simulink model "CiEngineController"  (R2026b)
undefined symbols (not defined in the file): CtrlEcuTs
libraries: autolibengctrlr x1
settings Model: Creator=The MathWorks, Inc.  LastModifiedBy=The MathWorks, Inc.

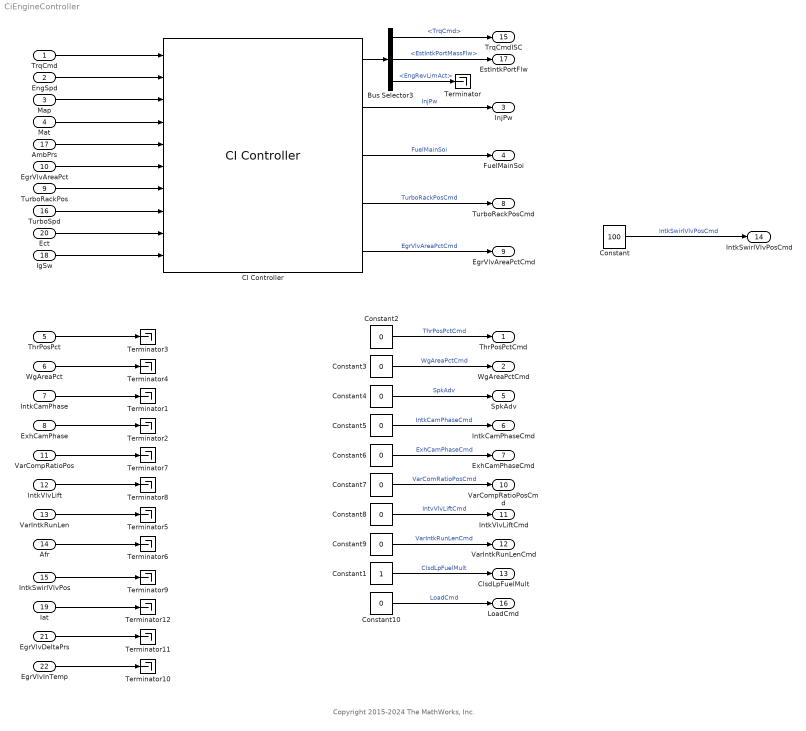
== system CiEngineController ==
  note: Copyright 2015-2024 The MathWorks, Inc.
  TrqCmd : Inport  OutDataTypeStr=double  Unit=N*m  PortDimensions=1
  EngSpd : Inport  Port=2  OutDataTypeStr=double  Unit=rpm  PortDimensions=1
  Map : Inport  Port=3  OutDataTypeStr=double  Unit=Pa  PortDimensions=1
  Mat : Inport  Port=4  OutDataTypeStr=double  Unit=K  PortDimensions=1
  ThrPosPct : Inport  Port=5  OutDataTypeStr=double  Unit=%  PortDimensions=1
  WgAreaPct : Inport  Port=6  OutDataTypeStr=double  Unit=%  PortDimensions=1
  IntkCamPhase : Inport  Port=7  OutDataTypeStr=double  Unit=deg  PortDimensions=1
  ExhCamPhase : Inport  Port=8  OutDataTypeStr=double  Unit=deg  PortDimensions=1
  TurboRackPos : Inport  Port=9  OutDataTypeStr=double  Unit=1  PortDimensions=1
  EgrVlvAreaPct : Inport  Port=10  OutDataTypeStr=double  Unit=%  PortDimensions=1
  VarCompRatioPos : Inport  Port=11  OutDataTypeStr=double  PortDimensions=1
  IntkVlvLift : Inport  Port=12  OutDataTypeStr=double  PortDimensions=1
  VarIntkRunLen : Inport  Port=13  OutDataTypeStr=double  PortDimensions=1
  Afr : Inport  Port=14  OutDataTypeStr=double  Unit=1  PortDimensions=1
  IntkSwirlVlvPos : Inport  Port=15  OutDataTypeStr=double  PortDimensions=1
  TurboSpd : Inport  Port=16  OutDataTypeStr=double  Unit=rpm  PortDimensions=1
  AmbPrs : Inport  Port=17  OutDataTypeStr=double  Unit=Pa  PortDimensions=1
  IgSw : Inport  Port=18  OutDataTypeStr=boolean  PortDimensions=1
  Iat : Inport  Port=19  OutDataTypeStr=double  Unit=K  PortDimensions=1
  Ect : Inport  Port=20  OutDataTypeStr=double  Unit=K  PortDimensions=1
  EgrVlvDeltaPrs : Inport  Port=21  OutDataTypeStr=double  Unit=Pa  PortDimensions=1
  EgrVlvInTemp : Inport  Port=22  OutDataTypeStr=double  Unit=K  PortDimensions=1
  Bus Selector3 : BusSelector  OutputSignals=TrqCmd,EstIntkPortMassFlw,EngRevLimAct
  CI Controller : autolibengctrlr/CI Controller  TrqEstOptionPopup=Torque Structure  f_egrcmd=CtrlEcuCIEgrCmd  f_egr_tq_bpt=CtrlEcuCIEgrTqBpt  f_egr_n_bpt=CtrlEcuCIEgrNBpt  f_rpcmd=CtrlEcuCIRpCmd  f_rp_tq_bpt=CtrlEcuCIRpTqBpt  f_rp_n_bpt=CtrlEcuCIRpNBpt  Sinj=PlntEngCISinj  afr_stoich=PlntEngAfrStoich  fuel_lhv=PlntEngDieselLhv  f_fcmd_tot=CtrlEcuCICmdTot  f_main_soi=CtrlEcuCIMainSoi  f_main_soi_f_bpt=CtrlEcuCIMainSoiFBpt  f_main_soi_n_bpt=CtrlEcuCIMainSoiNBpt  f_f_tot_tq_bpt=CtrlEcuCITotTqBpt  f_f_tot_n_bpt=CtrlEcuCITotNBpt  N_idle=CtrlEcuCINidle  Trq_idlecmd_enable=1  Trq_idlecmd_max=50  Kp_idle=0.1  Ki_idle=0.05  EngRevLim=CtrlEcuCIEngRevLim  ESSEnable=on  ESSExternalPortEnable=off  EngStopTime=CtrlEcuStopTime  CatLightOffTime=CtrlEcuCatLOff  Ts=CtrlEcuTs  NCyl=PlntEngCINCyl  Cps=PlntEngCICps  Vd=PlntEngCIVd  Rair=EnvRair  Pstd=EnvAbsPrs  Tstd=EnvAirTemp  f_nv=PlntEngCINv  f_nv_prs_bpt=PlntEngCINvPrsBpt  f_nv_n_bpt=PlntEngCINvNBpt  f_egr_stdflow=CtrlEcuCIEgrStdFlw  f_egr_stdflow_pr_bpt=CtrlEcuCIEgrStdFlwPrBpt  f_egr_stdflow_egrap_bpt=CtrlEcuCIEgrStdFlwEgrapBpt  f_turbo_pr=CtrlEcuCITrbPr  f_turbo_pr_stdflow_bpt=CtrlEcuCITrbPrStdFlwBpt  f_turbo_pr_corrspd_bpt=CtrlEcuCITrbPrCorrSpdBpt  f_turbo_pr_vgtposcorr=CtrlEcuCITrbPrVgtPosCorr  f_turbo_pr_vgtposcorr_bpt=CtrlEcuCITrbPrVgtPosCorBpt  f_tq_nf=PlntEngTqNf  f_tq_nf_f_bpt=PlntEngTqNfFBpt  f_tq_nf_n_bpt=PlntEngTqNfNBpt  f_tqs_f_bpt=PlntEngCIGIMepFuelBpt  f_tqs_n_bpt=PlntEngCIGIMepSpdBpt  f_tqs_mainsoi=PlntEngTqsMainSoi  f_tqs_map=PlntEngTqsMap  f_tqs_emap=PlntEngTqsEMap  f_tqs_mat=PlntEngTqsMat  f_tqs_o2pct=PlntEngTqsO2Pct  f_tqs_fuelpress=PlntEngTqsFuelPres  f_tqs_imepg=PlntEngCIGIMepMap  f_tqs_fmep=PlntEngTqsFMep  f_tqs_pmep=PlntEngTqsPMEP  f_tqs_fric_temp_mod=PlntEngTqsFrTmpMod  f_tqs_fric_temp_bpt=PlntEngTqsFrTmpBpt  f_tqs_mainsoi_eff=PlntEngTqsMainSoiEff  f_tqs_mainsoi_delta_bpt=PlntEngTqsMainSoiDeltaBpt  f_tqs_map_eff=PlntEngTqsMapEff  f_tqs_map_ratio_bpt=PlntEngTqsMapRatioBpt  f_tqs_lambda_bpt=PlntEngTqsLambdaBpt  f_tqs_mat_eff=PlntEngTqsMatEff  f_tqs_mat_delta_bpt=PlntEngTqsMatDeltaBpt  f_tqs_o2pct_eff=PlntEngTqsO2PctEff  f_tqs_o2pct_delta_bpt=PlntEngTqsO2PctDeltaBpt  f_tqs_fuelpress_eff=PlntEngTqsFuelPrsEff  f_tqs_fuelpress_delta_bpt=PlntEngTqsFuelPrsDeltaBpt  f_tqs_f_inj_type=PlntEngTqsInjType  f_tqs_imep_post_corr=PlntEngTqsImepPostCorr  f_tqs_f_post_sum_bpt=PlntEngTqsPostSumBpt  f_tqs_soi_post_cent_bpt=PlntEngTqsSoiPostCenBpt  f_tqs_f_burned_soi_limit=PlntEngTqsBurnedSoiLim  cp_exh=PlntEngCpExh  f_t_exh=CtrlEcuCITexh  f_t_exh_f_bpt=CtrlEcuCITexhFBpt  f_t_exh_n_bpt=CtrlEcuCITexhNBpt  f_tqs_exht=PlntEngTqsExhT  f_tqs_exht_mainsoi_eff=PlntEngTqsExhTMainSoiEff  f_tqs_exht_map_eff=PlntEngTqsExhTMapEff  f_tqs_exht_mat_eff=PlntEngTqsExhTMatEff  f_tqs_exht_o2pct_eff=PlntEngTqsExhTO2PctEff  f_tqs_exht_fuelpress_eff=PlntEngTqsExhTFuelPrsEff  f_tqs_exht_post_inj_wall_htc=PlntEngTqsExhTPstInjWHtc
  Constant : Constant  Value=100  SampleTime=-1
  Constant1 : Constant  SampleTime=-1
  Constant{2..10} (9 alike) : Constant  Value=0  SampleTime=-1
  Terminator{,1..12} (13 alike) : Terminator
  ThrPosPctCmd : Outport  OutDataTypeStr=double  Unit=%  PortDimensions=1  VectorParamsAs1DForOutWhenUnconnected=off
  WgAreaPctCmd : Outport  Port=2  OutDataTypeStr=double  Unit=%  PortDimensions=1  VectorParamsAs1DForOutWhenUnconnected=off
  InjPw : Outport  Port=3  OutDataTypeStr=double  Unit=ms  PortDimensions=1  VectorParamsAs1DForOutWhenUnconnected=off
  FuelMainSoi : Outport  Port=4  OutDataTypeStr=double  Unit=deg  PortDimensions=1  VectorParamsAs1DForOutWhenUnconnected=off
  SpkAdv : Outport  Port=5  OutDataTypeStr=double  Unit=deg  PortDimensions=1  VectorParamsAs1DForOutWhenUnconnected=off
  IntkCamPhaseCmd : Outport  Port=6  OutDataTypeStr=double  Unit=deg  PortDimensions=1  VectorParamsAs1DForOutWhenUnconnected=off
  ExhCamPhaseCmd : Outport  Port=7  OutDataTypeStr=double  Unit=deg  PortDimensions=1  VectorParamsAs1DForOutWhenUnconnected=off
  TurboRackPosCmd : Outport  Port=8  OutDataTypeStr=double  Unit=1  PortDimensions=1  VectorParamsAs1DForOutWhenUnconnected=off
  EgrVlvAreaPctCmd : Outport  Port=9  OutDataTypeStr=double  Unit=%  PortDimensions=1  VectorParamsAs1DForOutWhenUnconnected=off
  VarCompRatioPosCmd : Outport  Port=10  OutDataTypeStr=double  PortDimensions=1  VectorParamsAs1DForOutWhenUnconnected=off
  IntkVlvLiftCmd : Outport  Port=11  OutDataTypeStr=double  PortDimensions=1  VectorParamsAs1DForOutWhenUnconnected=off
  VarIntkRunLenCmd : Outport  Port=12  OutDataTypeStr=double  PortDimensions=1  VectorParamsAs1DForOutWhenUnconnected=off
  ClsdLpFuelMult : Outport  Port=13  OutDataTypeStr=double  Unit=1  PortDimensions=1  VectorParamsAs1DForOutWhenUnconnected=off
  IntkSwirlVlvPosCmd : Outport  Port=14  OutDataTypeStr=double  PortDimensions=1  VectorParamsAs1DForOutWhenUnconnected=off
  TrqCmdISC : Outport  Port=15  OutDataTypeStr=double  Unit=N*m  PortDimensions=1  VectorParamsAs1DForOutWhenUnconnected=off
  LoadCmd : Outport  Port=16  OutDataTypeStr=double  Unit=1  PortDimensions=1  VectorParamsAs1DForOutWhenUnconnected=off
  EstIntkPortFlw : Outport  Port=17  OutDataTypeStr=double  Unit=kg/s  PortDimensions=1  VectorParamsAs1DForOutWhenUnconnected=off
  wires:
  AmbPrs/1 -> CI Controller/5
  Map/1 -> CI Controller/3
  Mat/1 -> CI Controller/4
  IntkCamPhase/1 -> Terminator1/1
  ExhCamPhase/1 -> Terminator2/1
  CI Controller/1 -> Bus Selector3/1
  EngSpd/1 -> CI Controller/2
  Constant2/1 -> ThrPosPctCmd/1  "ThrPosPctCmd"
  TrqCmd/1 -> CI Controller/1
  CI Controller/4 -> TurboRackPosCmd/1  "TurboRackPosCmd"
  CI Controller/5 -> EgrVlvAreaPctCmd/1  "EgrVlvAreaPctCmd"
  Constant3/1 -> WgAreaPctCmd/1  "WgAreaPctCmd"
  Constant4/1 -> SpkAdv/1  "SpkAdv"
  Constant5/1 -> IntkCamPhaseCmd/1  "IntkCamPhaseCmd"
  Constant6/1 -> ExhCamPhaseCmd/1  "ExhCamPhaseCmd"
  Bus Selector3/2 -> EstIntkPortFlw/1  "<EstIntkPortMassFlw>"
  Constant10/1 -> LoadCmd/1  "LoadCmd"
  CI Controller/3 -> FuelMainSoi/1  "FuelMainSoi"
  EgrVlvAreaPct/1 -> CI Controller/6
  TurboRackPos/1 -> CI Controller/7
  TurboSpd/1 -> CI Controller/8
  CI Controller/2 -> InjPw/1  "InjPw"
  Constant7/1 -> VarCompRatioPosCmd/1  "VarComRatioPosCmd"
  Constant8/1 -> IntkVlvLiftCmd/1  "IntvVlvLiftCmd"
  Constant9/1 -> VarIntkRunLenCmd/1  "VarIntkRunLenCmd"
  Constant1/1 -> ClsdLpFuelMult/1  "ClsdLpFuelMult"
  Constant/1 -> IntkSwirlVlvPosCmd/1  "IntkSwirlVlvPosCmd"
  WgAreaPct/1 -> Terminator4/1
  ThrPosPct/1 -> Terminator3/1
  VarCompRatioPos/1 -> Terminator7/1
  IntkVlvLift/1 -> Terminator8/1
  Afr/1 -> Terminator6/1
  VarIntkRunLen/1 -> Terminator5/1
  IntkSwirlVlvPos/1 -> Terminator9/1
  Ect/1 -> CI Controller/9
  Iat/1 -> Terminator12/1
  EgrVlvInTemp/1 -> Terminator10/1
  EgrVlvDeltaPrs/1 -> Terminator11/1
  Bus Selector3/3 -> Terminator/1  "<EngRevLimAct>"
  IgSw/1 -> CI Controller/10
  Bus Selector3/1 -> TrqCmdISC/1  "<TrqCmd>"
